simulink model "c2f_workspace"  (R2019b)
settings: Solver=ode45  StartTime=0.0  StopTime=364  RelTol=1e-3  EnableMultiTasking=on
PreLoadFcn:
  | t = [0:364]';
  | load bangaloreTempsC;
  | tempData = [t TmaxC];
values from neighbouring files (symbols this model uses):
  TmaxC = [27.1111111111 27.7777777778 29.1111111111 30.2777777778 28.2222222222 29.1111111111 28.8888888889 26.7777777778 25.8888888889 30.2777777778 31.7777777778 30.5 ... (365 elements, 365x1)]    [bangaloreTempsC.mat]
settings Model: Creator=bbhattac  LastModifiedBy=khung
settings DataIOCC: LimitDataPoints=on  SaveFormat=Array  SignalLoggingSaveFormat=ModelDataLogs  ReturnWorkspaceOutputs=off
settings OptimizationCC: ExpressionDepthLimit=2147483647  LifeSpan=inf
settings DebuggingCC: UnderspecifiedInitializationDetection=Classic  MergeDetectMultiDrivingBlocksExec=none  SolverPrmCheckMsg=warning  FcnCallInpInsideContextMsg=warning  StateNameClashWarn=warning  SFUnexpectedBacktrackingDiag=warning  SFNoUnconditionalDefaultTransitionDiag=warning  SFExecutionAtInitializationDiag=none  ArithmeticOperatorsInVariantConditions=warning
settings HardwareCC: ProdBitPerPointer=32  ProdBitPerSizeT=32  ProdBitPerPtrDiffT=32  ProdLargestAtomicFloat=None  ProdIntDivRoundTo=Undefined  ProdEndianess=Unspecified  ProdWordSize=32  ProdHWDeviceType=32-bit Generic
settings ModelReferenceCC: PropagateSignalLabelsOutOfModel=off
settings SFSimCC: SimUseLocalCustomCode=off
settings RTWCC: RTWUseLocalCustomCode=off
settings CodeAppCC: StateflowObjectComments=on
settings GRTTargetCC: TargetLangStandard=C89/C90 (ANSI)  GeneratePreprocessorConditionals=Disable all  CombineOutputUpdateFcns=off  GRTInterface=on
settings ConfigComp: CovMetricSettings=dw  CovHtmlReporting=on  CovSaveCumulativeToWorkspaceVar=on  CovSaveSingleToWorkspaceVar=on  CovExternalEMLEnable=off

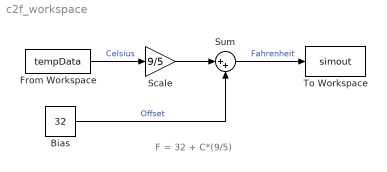
== system c2f_workspace ==
  note: F = 32 + C*(9/5)
  Bias : Constant  Value=32
  From Workspace : FromWorkspace  VariableName=tempData  SampleTime=0
  Scale : Gain  Gain=9/5
  Sum : Sum  Inputs=|++
  To Workspace : ToWorkspace  VariableName=simout  SaveFormat=Structure  SampleTime=-1
  wires:
  From Workspace/1 -> Scale/1  "Celsius"
  Scale/1 -> Sum/1
  Bias/1 -> Sum/2  "Offset"
  Sum/1 -> To Workspace/1  "Fahrenheit"
